simulink model "NLPIDVersion2"  (Simulink 7.3)
settings: Solver=ode5  StartTime=0.0  StopTime=inf  FixedStep=0.1  RelTol=1e-3
undefined symbols (not defined in the file): eta1_0_real, v1_0_real, velocitySatValues1
libraries: dspmtrx3 x16, simulink x14, dspindex x5, marine_gnc x4, simulink_extras x1, dspinverses x1
(part 1 of 4)
settings Model: Creator=Dinh  LastModifiedBy=mcl  BufferReuse=off
settings DataIOCC: LimitDataPoints=off  SaveOutput=off  SaveTime=off
settings OptimizationCC: BlockReduction=off  BooleanDataType=off  ConditionallyExecuteInputs=off  OptimizeBlockIOStorage=off  BufferReuse=off  ExpressionFolding=off  LocalBlockOutputs=off  SimCompilerOptimization=On
settings SFSimCC: SimBuildMode=sf_nonincremental_build
settings RTWCC: SystemTargetFile=nidll.tlc  TemplateMakefile=nidll_vc.tmf  Description=NI Real-Time Target for Release 2007b or later  ProcessScript=nidll_make_rtw_hook
settings STFCustomTargetCC: MatFileLogging=on  SystemTargetFile=nidll.tlc

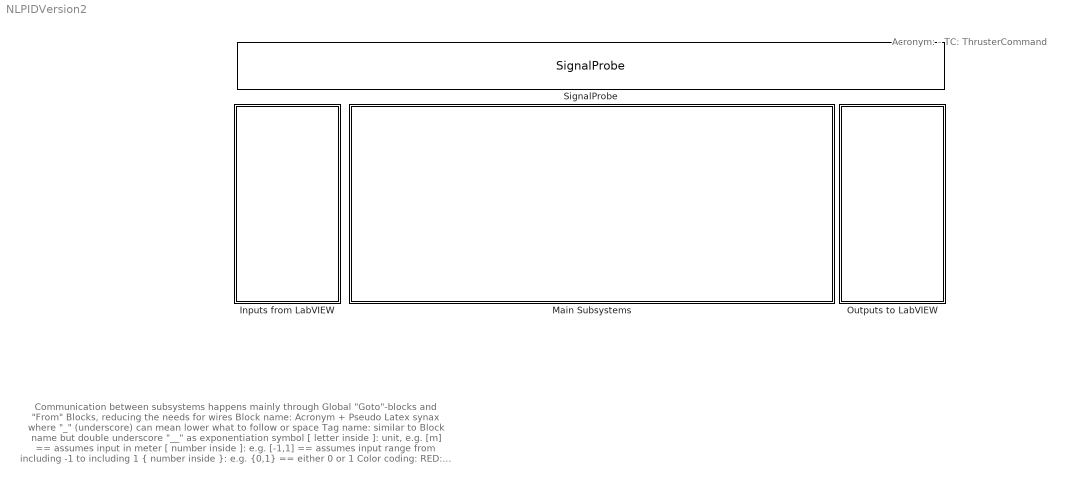
== system NLPIDVersion2 ==
  note: Communication between subsystems happens mainly through Global "Goto"-blocks and "From" Blocks,
      | reducing the needs for wires
      |
      | Block name: Acronym + Pseudo Latex synax where "_" (underscore) can mean lower what to follow or space
      | Tag name: similar to Block name but double underscore "__" as exponentiation symbol
      |
      | [ letter inside ]: unit, e.g. [m] == assumes input in meter
      | [ number inside ]: e.g. [-1,1] == assumes input range from including -1 to including 1
      | { number inside }:  e.g. {0,1} == either 0 or 1
      |
      | Color coding:
      | RED: Sinks (output ports, terminators, to workspace blocks, etc.)
      | GREEN Sources (inputs ports, constants, etc.)
      | CYAN: Memory blocks: Integrators, unit delays, memory, transfer functions, state space blocks, etc
      | GRAY: Logics blocks: Logic action ports, subsystem enable, etc.
      | ORANGE: GOTO blocks
      | MAGENTA: FROM blocks
      | YELLOW: All remaining blocks,
  note: Acronym:
      | - TC: ThrusterCommand
  Inputs from LabVIEW : Subsystem
  Main Subsystems : Subsystem
  Outputs to LabVIEW : Subsystem
  SignalProbe : S-Function  Description=Use this block with SIT.  FunctionName=SignalProbe  Parameters=1  EnableBusSupport=off
      settings: PreSaveFcn=NISIT_ModelVars;
      mask Description: The LabVIEW Simulation Interface Toolkit uses the SignalProbe block to probe the signals in the model. The SignalProbe block must be on the top level of the model hierarchy. You can have only one SignalProbe block per model file. Do not rename the SignalProbe block. Do not change the name of another model block to SignalProbe.

== system NLPIDVersion2/Inputs from LabVIEW ==
  Control Input Selector : Constant  Value=0
  Control Mode Selector : Constant  Value=0
  Enable CSE1 : Constant  Value=0
  Linear Simulator : Subsystem
  Path : Subsystem
  PlayStation3 : Subsystem
  Setpoint : Subsystem
  ctrl1: Dynamic Positioning : Subsystem
  ctrl2: LOS LgV backstepping II : Subsystem
  tag scope: controlInputSelector=global, controlModeSelector=global, enableCSE1=global
  wires:
  Control Mode Selector/1 -> [controlModeSelector]
  Control Input Selector/1 -> [controlInputSelector]
  Enable CSE1/1 -> [enableCSE1]

== system NLPIDVersion2/Main Subsystems ==
  C/S Enterprise 1 Matrices : Subsystem
  Control : Subsystem
  Data logging : Subsystem
  Guidance : Subsystem
  Naviagation : Subsystem
  Plant : Subsystem

== system NLPIDVersion2/Outputs to LabVIEW ==
  note: Gain blocks in this subsystem, functions as output ports for linking LabVIEW indicators through SIT Connection Manager
  Battery Voltage : Subsystem
  Command : Subsystem
  Mux9 : Mux  Inputs=2
  Naviagtion : Subsystem
  Visualization : Subsystem
  tag scope: eta_d=global
  wires:
  [pd] -> Mux9/1
  [psid] -> Mux9/2
  Mux9/1 -> [eta_d]

== system NLPIDVersion2/Inputs from LabVIEW/Linear Simulator ==
  note: Enable Linear Simulator: Activation
      | Reset Linear Simulator integrator: Reset
      | Initial u: Initial speed in surge
      | Initial v: Initial speed in sway
      | Initial r: Initial speed in yaw
      | Initial x: Initial position in surge
      | Initial y: Initial position in sway
      | Initial psi: Initial heading
  Enable Linear Simulator : Constant  Value=0
  Initial psi [rad] : Constant  Value=0  OutDataType=fixdt(1, 16)  OutScaling=2^0
  Initial r [rad/s] : Constant  Value=0  OutDataType=fixdt(1, 16)  OutScaling=2^0
  Initial u [m/s] : Constant  Value=0  OutDataType=fixdt(1, 16)  OutScaling=2^0
  Initial v [m/s] : Constant  Value=0  OutDataType=fixdt(1, 16)  OutScaling=2^0
  Initial x [m] : Constant  Value=0  OutDataType=fixdt(1, 16)  OutScaling=2^0
  Initial y [m] : Constant  Value=0  OutDataType=fixdt(1, 16)  OutScaling=2^0
  Mux : Mux  Inputs=3
  Mux1 : Mux  Inputs=3
  Reset Linear Simulator integrator : Constant  Value=0
  tag scope: LS_Enable=global, LS_Initial_eta=global, LS_Initial_nu=global, LS_Reset=global
  wires:
  Enable Linear Simulator/1 -> [LS_Enable]
  Reset Linear Simulator integrator/1 -> [LS_Reset]
  Mux/1 -> [LS_Initial_nu]
  Initial r [rad/s]/1 -> Mux/3
  Initial v [m/s]/1 -> Mux/2
  Initial u [m/s]/1 -> Mux/1
  Mux1/1 -> [LS_Initial_eta]
  Initial psi [rad]/1 -> Mux1/3
  Initial y [m]/1 -> Mux1/2
  Initial x [m]/1 -> Mux1/1

== system NLPIDVersion2/Inputs from LabVIEW/Path ==
  note: u_d: Desired surge speed of vessel
      | Path Selector: Workaround parameter for switching between linear path(==0) and ellipse path(==1)
      | x_dmax: Upper limit of desired x-ooordinate
      | x_dmin: Lower limit of desired x-coordiante
      | y_dmax: Upper limit of desired y-ooordinate
      | y_dmin: Lower limit of desired y-coordiante
      | Delta: Lookahead distance for LOS guidance
      | my: Gradient path minimizing tuning value
  Delta [m] : Constant  Value=2  OutDataType=fixdt(1, 16)  OutScaling=2^0
  Ellipse : Subsystem
  Linear : Subsystem
  Path Selector  [-] : Constant  Value=0
  my [-] : Constant  Value=10  OutDataType=fixdt(1, 16)  OutScaling=2^0
  u_d [m] : Constant  Value=0.15  OutDataType=fixdt(1, 16)  OutScaling=2^0
  x_dmax [m] : Constant  Value=40
  x_dmin [m] : Constant  Value=-40
  y_dmax [m] : Constant  Value=7
  y_dmin [m] : Constant  Value=-7
  tag scope: Delta=global, my=global, pathSelector=global, ud=global, xdmax=global, xdmin=global, ydmax=global, ydmin=global
  wires:
  u_d [m]/1 -> [ud]  "Desired speed [m/s]"
  Delta [m]/1 -> [Delta]  "Lookahead distance [m]"
  my [-]/1 -> [my]  "s tuning parameter"
  Path Selector  [-]/1 -> [pathSelector]  "chosen path {0,1}"
  x_dmax [m]/1 -> [xdmax]
  x_dmin [m]/1 -> [xdmin]
  y_dmax [m]/1 -> [ydmax]
  y_dmin [m]/1 -> [ydmin]

== system NLPIDVersion2/Inputs from LabVIEW/PlayStation3 ==
  note: Postive Y-axis of analog sticks points up (in the direction of the shoulder buttons)
      | Postive X-axis of analog sticks points to the right (in the direction of Triange, Circle, X and Square buttons)
      |
      | AS_LX: PS3 Analog Stick Left X-postition
      | AS_LY: PS3 Analog Stick Left Y-postition
      | AS_RX: PS3 Analog Stick Right X-postition
      | AS_RY: PS3 Analog Stick Right Y-postition
      | L2: PS3 bottom left sholderbutton
      | R2: PS3 bottom right shoulderbotton
      | PS3_BT_Power: PS3 command bow thruster power setpoint
      | PS3 _VSP_speed: PS3 command Voith Schneider Propeller speed
  "AS_LX [-] " : Constant  Value=0
  AS_LY [-] : Constant  Value=0
  AS_RX [-] : Constant  Value=0
  AS_RY [-] : Constant  Value=0
  L2 [-] : Constant  Value=0
  PS3_BT_Power  [-] : Constant  Value=0
  PS3_VSP_Speed  [-] : Constant  Value=0
  R2 [-] : Constant  Value=0
  ScalingLX : Gain  Gain=1/32767
  ScalingLY : Gain  Gain=1/32767
  ScalingRY : Gain  Gain=1/32767
  Scaling_RX : Gain  Gain=1/32767
  tag scope: PS3_AS_LX=global, PS3_AS_LY=global, PS3_AS_RX=global, PS3_AS_RY=global, PS3_BT_Power=global, PS3_L2=global, PS3_R2=global, PS3_VSP_Speed=global
  wires:
  PS3_VSP_Speed  [-]/1 -> [PS3_VSP_Speed]  "Voith Schnider Propeller Speed"
  PS3_BT_Power  [-]/1 -> [PS3_BT_Power]  "Bow Thruster Power"
  "AS_LX [-] "/1 -> ScalingLX/1  "x-position of left analog stick [-32767,32767]"
  ScalingLX/1 -> [PS3_AS_LX]  "x-position of left analog stick [-1,1]"
  AS_LY [-]/1 -> ScalingLY/1  "y-position of left analog stick [-32767,32767]"
  ScalingLY/1 -> [PS3_AS_LY]  "y-position of left analog stick [-1,1]"
  AS_RX [-]/1 -> Scaling_RX/1  "x-position of right analog stick  [-32767,32767]"
  Scaling_RX/1 -> [PS3_AS_RX]  "x-position of right analog stick  [-1,1]"
  ScalingRY/1 -> [PS3_AS_RY]  "y-position of right analog stick [-1,1]"
  AS_RY [-]/1 -> ScalingRY/1  "y-position of right analog stick [-32767,32767]"
  L2 [-]/1 -> [PS3_L2]  "L2 Button [-1,0]"
  R2 [-]/1 -> [PS3_R2]  "R2 Button [0,1]"

== system NLPIDVersion2/Inputs from LabVIEW/Setpoint ==
  Degrees to Radians : simulink_extras/Transformations/Degrees to Radians  SystemSampleTime=-1
  Mux : Mux  Inputs=3
  setpointpsi [deg] : Constant  Value=0
  setpointx [m] : Constant  Value=0
  setpointy [m] : Constant  Value=0
  tag scope: setpoint=global
  wires:
  Mux/1 -> [setpoint]
  setpointx [m]/1 -> Mux/1
  setpointy [m]/1 -> Mux/2
  setpointpsi [deg]/1 -> Degrees to Radians/1
  Degrees to Radians/1 -> Mux/3

== system NLPIDVersion2/Inputs from LabVIEW/ctrl1: Dynamic Positioning ==
  Kd : Subsystem
  Ki : Subsystem
  Kp : Subsystem
  "ctrl1 Reset Integrator " : Constant  Value=0
  ctrl1Kdpsi : Constant  Value=5
  ctrl1Kdx : Constant  Value=50
  ctrl1Kdy : Constant  Value=30
  ctrl1Kipsi : Constant  Value=0
  ctrl1Kix : Constant  Value=0
  ctrl1Kiy : Constant  Value=0
  ctrl1Kppsi : Constant  Value=0.5*3
  ctrl1Kpx : Constant  Value=2*1.5*2
  ctrl1Kpy : Constant  Value=2*10*2
  tag scope: ctrl1Reset=global
  wires:
  "ctrl1 Reset Integrator "/1 -> [ctrl1Reset]
  ctrl1Kpx/1 -> Kp/1(11)
  ctrl1Kpy/1 -> Kp/2(22)
  ctrl1Kppsi/1 -> Kp/3(33)
  ctrl1Kdx/1 -> Kd/1(11)
  ctrl1Kdy/1 -> Kd/2(22)
  ctrl1Kdpsi/1 -> Kd/3(33)
  ctrl1Kix/1 -> Ki/1(11)
  ctrl1Kiy/1 -> Ki/2(22)
  ctrl1Kipsi/1 -> Ki/3(33)

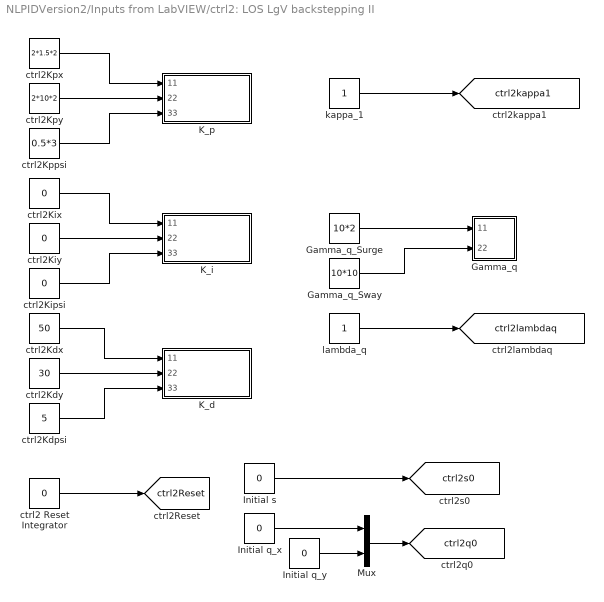
== system NLPIDVersion2/Inputs from LabVIEW/ctrl2: LOS LgV backstepping II ==
  Gamma_q : Subsystem
  Gamma_q_Surge : Constant  Value=10*2
  Gamma_q_Sway : Constant  Value=10*10
  Initial q_x : Constant  Value=0  OutDataType=fixdt(1, 16)  OutScaling=2^0
  Initial q_y : Constant  Value=0  OutDataType=fixdt(1, 16)  OutScaling=2^0
  Initial s : Constant  Value=0  OutDataType=fixdt(1, 16)  OutScaling=2^0
  K_d : Subsystem
  K_i : Subsystem
  K_p : Subsystem
  Mux : Mux  Inputs=2
  "ctrl2 Reset Integrator " : Constant  Value=0
  ctrl2Kdpsi : Constant  Value=5
  ctrl2Kdx : Constant  Value=50
  ctrl2Kdy : Constant  Value=30
  ctrl2Kipsi : Constant  Value=0
  ctrl2Kix : Constant  Value=0
  ctrl2Kiy : Constant  Value=0
  ctrl2Kppsi : Constant  Value=0.5*3
  ctrl2Kpx : Constant  Value=2*1.5*2
  ctrl2Kpy : Constant  Value=2*10*2
  kappa_1 : Constant
  lambda_q : Constant
  tag scope: ctrl2Reset=global, ctrl2kappa1=global, ctrl2lambdaq=global, ctrl2q0=global, ctrl2s0=global
  wires:
  ctrl2Kpx/1 -> K_p/1(11)
  ctrl2Kpy/1 -> K_p/2(22)
  ctrl2Kppsi/1 -> K_p/3(33)
  ctrl2Kdx/1 -> K_d/1(11)
  ctrl2Kdy/1 -> K_d/2(22)
  ctrl2Kdpsi/1 -> K_d/3(33)
  ctrl2Kix/1 -> K_i/1(11)
  ctrl2Kiy/1 -> K_i/2(22)
  ctrl2Kipsi/1 -> K_i/3(33)
  Gamma_q_Surge/1 -> Gamma_q/1(11)
  Gamma_q_Sway/1 -> Gamma_q/2(22)
  kappa_1/1 -> [ctrl2kappa1]
  lambda_q/1 -> [ctrl2lambdaq]
  Initial q_x/1 -> Mux/1
  Initial q_y/1 -> Mux/2
  Initial s/1 -> [ctrl2s0]
  Mux/1 -> [ctrl2q0]
  "ctrl2 Reset Integrator "/1 -> [ctrl2Reset]

== system NLPIDVersion2/Main Subsystems/C/S Enterprise 1 Matrices ==
  Inertia matrix : Subsystem
  Linear hydrodynamic dampning matrix : Subsystem
  Thruster configuration matrix : Subsystem
  tag scope: B=global, DL=global, M=global
  wires:
  Inertia matrix/1(M) -> [M]
  Linear hydrodynamic dampning matrix/1(D_L) -> [DL]
  Thruster configuration matrix/1(B) -> [B]

== system NLPIDVersion2/Main Subsystems/Control ==
  Control Switch : Subsystem
  DP control : Subsystem
  Nonlinear PID : Subsystem
  PS3 u input control : Subsystem
      settings: MinAlgLoopOccurrences=on
  Thruster allocation : Subsystem

== system NLPIDVersion2/Main Subsystems/Data logging ==
  note: Data logging:
      | - Create a file named CSE1_data.mat in CRIO
      | - Top row contains timestamp run-time
      | Rows contain values of the vector sent into the block at timestamp
      | -Row 1: Time since simulation start
      | -Row 2: Selected navigation system, 0 == QS, 1 == LS
      | -Row 3: Error signal from Qualisys
      | -Row 4: Residual from Qualisys
      | -Row 5 to 7: etadot, col ( xdot, ydot, psidot)
      | -Row 8 to 10: eta, col (x, y, psi)
      | -Row 11 to 13: nu, col (u, v, r)
      | -Row 14 to 16: DP eta_d, col(x_d_DP, y_d_DP, psi_d_DP)
      | -Row 17 to 19: chi, col( q_x, q_y, psi_los)
      | -Row 20: Selected path, 0 == Ellipse, 1 = Linear
      | -Row 21 to 23: Path eta_d, col(x_d_path, y_d_path, psi_d_path)
      | -Row 24: u_d
      | -Row: 25: v_s
      | -Row 26: s
      | -Row 27: Selected control system
      | -Row 28 to 34: thruster setting, ( u_1, u_2, u_3, u_4. u_5, BT_limit, VSP_limit)
      | -Row 35 to 37: tau, col( X, Y, N)
      | -Row 38 to 39: omega_qx, omega_qy
  Mux2 : Mux  Inputs=17
  To File : ToFile  Filename=Template_data.mat  MatrixName=Template_data
  wires:
  Mux2/1 -> To File/1
  [controlInputSelector] -> Mux2/1
  [QTM_Error] -> Mux2/2
  [QTM_Residual] -> Mux2/3
  [etadot] -> Mux2/4
  [eta] -> Mux2/5
  [nu] -> Mux2/6
  [setpoint] -> Mux2/7
  [chi] -> Mux2/8
  [pathSelector] -> Mux2/9
  [eta_d] -> Mux2/10
  [ud] -> Mux2/11
  [vs] -> Mux2/12
  [s] -> Mux2/13
  [controlModeSelector] -> Mux2/14
  [ThrusterSetting] -> Mux2/15
  [tau] -> Mux2/16
  [omegaq] -> Mux2/17

== system NLPIDVersion2/Main Subsystems/Guidance ==
  Line-Of-Sight Path-Following : Subsystem

== system NLPIDVersion2/Main Subsystems/Naviagation ==
  Input from SIT : Subsystem
  Navigation Switch : Subsystem

== system NLPIDVersion2/Main Subsystems/Plant ==
  CSE1 actuator : Subsystem
  Inverse : Product  Inputs=/  Multiplication=Matrix(*)
  Linear Simulator : Subsystem
      settings: MinAlgLoopOccurrences=on
  Thruster setting workaround : Subsystem
  saturation : Subsystem
  tag scope: LS_eta=global, LS_etadot=global, LS_nu=global
  wires:
  [enableCSE1] -> CSE1 actuator/Enable
  [LS_Enable] -> Linear Simulator/Enable
  saturation/1(sat_tau) -> Linear Simulator/1(tau)
  [tau] -> saturation/1(tau)
  Linear Simulator/1(eta_hil) -> [LS_eta]
  Linear Simulator/2(nu_hil) -> [LS_nu]
  Linear Simulator/3(etadot_hil) -> [LS_etadot]
  [M] -> Inverse/1
  Inverse/1 -> Linear Simulator/2(M_inv)
  [DL] -> Linear Simulator/3(D_L)
  [LS_Reset] -> Linear Simulator/4(Reset)
  [LS_Initial_eta] -> Linear Simulator/5(eta_0)
  [LS_Initial_nu] -> Linear Simulator/6(nu_0)
  [TC] -> Thruster setting workaround/1(TC)
  [ThrusterSetting] -> CSE1 actuator/1(Thurster setting)

== system NLPIDVersion2/Outputs to LabVIEW/Battery Voltage ==
  note: Main battery is multipled by 2, since the voltage is halfed at measuring point
  Battery Bow Thruster : Gain  ParameterDataType=fixdt(1, 16)  ParameterScaling=2^0  OutDataType=fixdt(1, 16)  OutScaling=2^0
  Battery Main : Gain  Gain=2  ParameterDataType=fixdt(1, 16)  ParameterScaling=2^0  OutDataType=fixdt(1, 16)  OutScaling=2^0
  Battery Servo : Gain  ParameterDataType=fixdt(1, 16)  ParameterScaling=2^0  OutDataType=fixdt(1, 16)  OutScaling=2^0
  Terminator Bow Thruster Battery : Terminator
  Terminator Main Battery : Terminator
  Terminator Servo Battery : Terminator
  wires:
  [Battery_BT] -> Battery Bow Thruster/1
  Battery Bow Thruster/1 -> Terminator Bow Thruster Battery/1
  [Battery_Servo] -> Battery Servo/1
  Battery Servo/1 -> Terminator Servo Battery/1
  [Battery_Main] -> Battery Main/1
  Battery Main/1 -> Terminator Main Battery/1

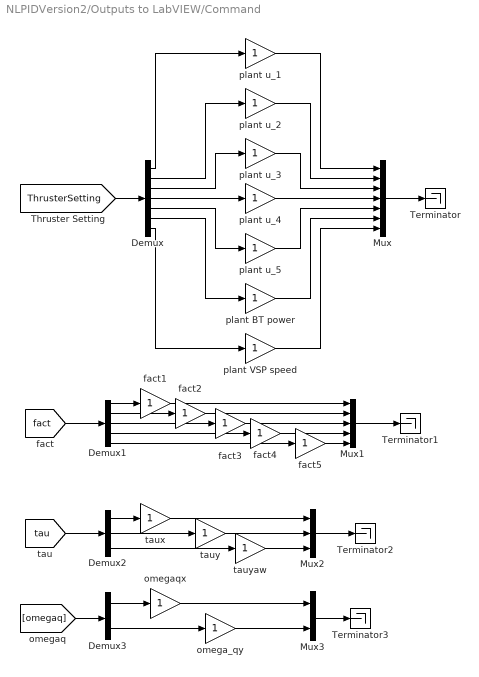
== system NLPIDVersion2/Outputs to LabVIEW/Command ==
  Demux : Demux  Outputs=7
  Demux1 : Demux  Outputs=5
  Demux2 : Demux  Outputs=3
  Demux3 : Demux  Outputs=2
  Mux : Mux  Inputs=7
  Mux1 : Mux  Inputs=5
  Mux2 : Mux  Inputs=3
  Mux3 : Mux  Inputs=2
  Terminator{,1..3} (4 alike) : Terminator
  fact{1..5} (5 alike) : Gain  ParameterDataType=fixdt(1, 16)  ParameterScaling=2^0  OutDataType=fixdt(1, 16)  OutScaling=2^0
  omega_qy : Gain  ParameterDataType=fixdt(1, 16)  ParameterScaling=2^0  OutDataType=fixdt(1, 16)  OutScaling=2^0
  omegaqx : Gain  ParameterDataType=fixdt(1, 16)  ParameterScaling=2^0  OutDataType=fixdt(1, 16)  OutScaling=2^0
  plant BT power : Gain  ParameterDataType=fixdt(1, 16)  ParameterScaling=2^0  OutDataType=fixdt(1, 16)  OutScaling=2^0
  plant VSP speed : Gain  ParameterDataType=fixdt(1, 16)  ParameterScaling=2^0  OutDataType=fixdt(1, 16)  OutScaling=2^0
  plant u_{1..5} (5 alike) : Gain  ParameterDataType=fixdt(1, 16)  ParameterScaling=2^0  OutDataType=fixdt(1, 16)  OutScaling=2^0
  taux : Gain  ParameterDataType=fixdt(1, 16)  ParameterScaling=2^0  OutDataType=fixdt(1, 16)  OutScaling=2^0
  tauy : Gain  ParameterDataType=fixdt(1, 16)  ParameterScaling=2^0  OutDataType=fixdt(1, 16)  OutScaling=2^0
  tauyaw : Gain  ParameterDataType=fixdt(1, 16)  ParameterScaling=2^0  OutDataType=fixdt(1, 16)  OutScaling=2^0
  wires:
  Demux/1 -> plant u_1/1
  Demux/2 -> plant u_2/1
  Demux/3 -> plant u_3/1
  Demux/4 -> plant u_4/1
  plant u_4/1 -> Mux/4
  plant u_1/1 -> Mux/1
  plant u_2/1 -> Mux/2
  plant u_3/1 -> Mux/3
  Demux/5 -> plant u_5/1
  Demux/6 -> plant BT power/1
  Demux/7 -> plant VSP speed/1
  plant u_5/1 -> Mux/5
  plant BT power/1 -> Mux/6
  plant VSP speed/1 -> Mux/7
  Mux/1 -> Terminator/1
  [ThrusterSetting] -> Demux/1
  fact1/1 -> Mux1/1
  fact2/1 -> Mux1/2
  fact3/1 -> Mux1/3
  fact4/1 -> Mux1/4
  fact5/1 -> Mux1/5
  Demux1/1 -> fact1/1
  Demux1/2 -> fact2/1
  Demux1/3 -> fact3/1
  Demux1/4 -> fact4/1
  Demux1/5 -> fact5/1
  [fact] -> Demux1/1
  Demux2/1 -> taux/1
  Demux2/2 -> tauy/1
  Demux2/3 -> tauyaw/1
  taux/1 -> Mux2/1
  tauy/1 -> Mux2/2
  tauyaw/1 -> Mux2/3
  Mux1/1 -> Terminator1/1
  Mux2/1 -> Terminator2/1
  [tau] -> Demux2/1
  Demux3/1 -> omegaqx/1
  Demux3/2 -> omega_qy/1
  omegaqx/1 -> Mux3/1
  omega_qy/1 -> Mux3/2
  Mux3/1 -> Terminator3/1
  [omegaq] -> Demux3/1

== system NLPIDVersion2/Outputs to LabVIEW/Naviagtion ==
  CSE1_r [deg/s] : Gain  Gain=180/pi  ParameterDataType=fixdt(1, 16)  ParameterScaling=2^0  OutDataType=fixdt(1, 16)  OutScaling=2^0
  CSE1_u [m/s] : Gain  ParameterDataType=fixdt(1, 16)  ParameterScaling=2^0  OutDataType=fixdt(1, 16)  OutScaling=2^0
  CSE1_v [m/s] : Gain  ParameterDataType=fixdt(1, 16)  ParameterScaling=2^0  OutDataType=fixdt(1, 16)  OutScaling=2^0
  Demux4 : Demux  Outputs=3
  Mux4 : Mux  Inputs=3
  Terminator3 : Terminator
  wires:
  CSE1_v [m/s]/1 -> Mux4/2
  CSE1_r [deg/s]/1 -> Mux4/3
  CSE1_u [m/s]/1 -> Mux4/1
  Demux4/3 -> CSE1_r [deg/s]/1
  Demux4/2 -> CSE1_v [m/s]/1
  Demux4/1 -> CSE1_u [m/s]/1
  Mux4/1 -> Terminator3/1
  [nu] -> Demux4/1

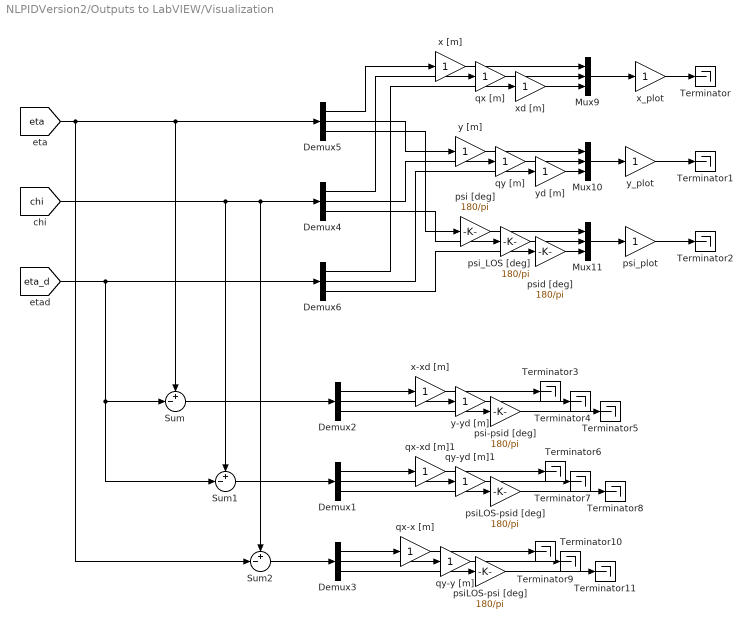
== system NLPIDVersion2/Outputs to LabVIEW/Visualization ==
  Demux{1..6} (6 alike) : Demux  Outputs=3
  Mux10 : Mux  Inputs=3
  Mux11 : Mux  Inputs=3
  Mux9 : Mux  Inputs=3
  Sum : Sum  Inputs=+-|  OutDataType=fixdt(1, 16)  OutScaling=2^0
  Sum1 : Sum  Inputs=+-|  OutDataType=fixdt(1, 16)  OutScaling=2^0
  Sum2 : Sum  Inputs=+-|  OutDataType=fixdt(1, 16)  OutScaling=2^0
  Terminator{,1..11} (12 alike) : Terminator
  psi [deg] : Gain  Gain=180/pi  ParameterDataType=fixdt(1, 16)  ParameterScaling=2^0  OutDataType=fixdt(1, 16)  OutScaling=2^0
  psi-psid [deg] : Gain  Gain=180/pi  ParameterDataType=fixdt(1, 16)  ParameterScaling=2^0  OutDataType=fixdt(1, 16)  OutScaling=2^0
  psiLOS-psi [deg] : Gain  Gain=180/pi  ParameterDataType=fixdt(1, 16)  ParameterScaling=2^0  OutDataType=fixdt(1, 16)  OutScaling=2^0
  psiLOS-psid [deg] : Gain  Gain=180/pi  ParameterDataType=fixdt(1, 16)  ParameterScaling=2^0  OutDataType=fixdt(1, 16)  OutScaling=2^0
  psi_LOS [deg] : Gain  Gain=180/pi  ParameterDataType=fixdt(1, 16)  ParameterScaling=2^0  OutDataType=fixdt(1, 16)  OutScaling=2^0
  psi_plot : Gain  ParameterDataType=fixdt(1, 16)  ParameterScaling=2^0  OutDataType=fixdt(1, 16)  OutScaling=2^0
  psid [deg] : Gain  Gain=180/pi  ParameterDataType=fixdt(1, 16)  ParameterScaling=2^0  OutDataType=fixdt(1, 16)  OutScaling=2^0
  qx [m] : Gain  ParameterDataType=fixdt(1, 16)  ParameterScaling=2^0  OutDataType=fixdt(1, 16)  OutScaling=2^0
  qx-x [m] : Gain  ParameterDataType=fixdt(1, 16)  ParameterScaling=2^0  OutDataType=fixdt(1, 16)  OutScaling=2^0
  qx-xd [m]1 : Gain  ParameterDataType=fixdt(1, 16)  ParameterScaling=2^0  OutDataType=fixdt(1, 16)  OutScaling=2^0
  qy [m] : Gain  ParameterDataType=fixdt(1, 16)  ParameterScaling=2^0  OutDataType=fixdt(1, 16)  OutScaling=2^0
  qy-y [m] : Gain  ParameterDataType=fixdt(1, 16)  ParameterScaling=2^0  OutDataType=fixdt(1, 16)  OutScaling=2^0
  qy-yd [m]1 : Gain  ParameterDataType=fixdt(1, 16)  ParameterScaling=2^0  OutDataType=fixdt(1, 16)  OutScaling=2^0
  x [m] : Gain  ParameterDataType=fixdt(1, 16)  ParameterScaling=2^0  OutDataType=fixdt(1, 16)  OutScaling=2^0
  x-xd [m] : Gain  ParameterDataType=fixdt(1, 16)  ParameterScaling=2^0  OutDataType=fixdt(1, 16)  OutScaling=2^0
  x_plot : Gain  ParameterDataType=fixdt(1, 16)  ParameterScaling=2^0  OutDataType=fixdt(1, 16)  OutScaling=2^0
  xd [m] : Gain  ParameterDataType=fixdt(1, 16)  ParameterScaling=2^0  OutDataType=fixdt(1, 16)  OutScaling=2^0
  y [m] : Gain  ParameterDataType=fixdt(1, 16)  ParameterScaling=2^0  OutDataType=fixdt(1, 16)  OutScaling=2^0
  y-yd [m] : Gain  ParameterDataType=fixdt(1, 16)  ParameterScaling=2^0  OutDataType=fixdt(1, 16)  OutScaling=2^0
  y_plot : Gain  ParameterDataType=fixdt(1, 16)  ParameterScaling=2^0  OutDataType=fixdt(1, 16)  OutScaling=2^0
  yd [m] : Gain  ParameterDataType=fixdt(1, 16)  ParameterScaling=2^0  OutDataType=fixdt(1, 16)  OutScaling=2^0
  wires:
  Demux5/1 -> x [m]/1
  Demux4/1 -> qx [m]/1
  Demux6/1 -> xd [m]/1
  Demux5/2 -> y [m]/1
  Demux4/2 -> qy [m]/1
  Demux6/2 -> yd [m]/1
  Demux5/3 -> psi [deg]/1
  Demux4/3 -> psi_LOS [deg]/1
  Demux6/3 -> psid [deg]/1
  Mux9/1 -> x_plot/1
  Mux10/1 -> y_plot/1
  Mux11/1 -> psi_plot/1
  x_plot/1 -> Terminator/1
  x [m]/1 -> Mux9/1
  qx [m]/1 -> Mux9/2
  xd [m]/1 -> Mux9/3
  y [m]/1 -> Mux10/1
  qy [m]/1 -> Mux10/2
  yd [m]/1 -> Mux10/3
  psi [deg]/1 -> Mux11/1
  psi_LOS [deg]/1 -> Mux11/2
  psid [deg]/1 -> Mux11/3
  y_plot/1 -> Terminator1/1
  psi_plot/1 -> Terminator2/1
  [eta] -> Demux5/1, Sum/1, Sum2/2
  [chi] -> Sum1/1, Demux4/1, Sum2/1
  [eta_d] -> Demux6/1, Sum/2, Sum1/2
  Sum/1 -> Demux2/1
  Sum1/1 -> Demux1/1
  Sum2/1 -> Demux3/1
  Demux2/1 -> x-xd [m]/1
  Demux2/2 -> y-yd [m]/1
  Demux2/3 -> psi-psid [deg]/1
  Demux1/1 -> qx-xd [m]1/1
  Demux1/2 -> qy-yd [m]1/1
  Demux1/3 -> psiLOS-psid [deg]/1
  Demux3/2 -> qy-y [m]/1
  Demux3/3 -> psiLOS-psi [deg]/1
  Demux3/1 -> qx-x [m]/1
  x-xd [m]/1 -> Terminator3/1
  y-yd [m]/1 -> Terminator4/1
  psi-psid [deg]/1 -> Terminator5/1
  qy-yd [m]1/1 -> Terminator7/1
  psiLOS-psid [deg]/1 -> Terminator8/1
  qx-xd [m]1/1 -> Terminator6/1
  qy-y [m]/1 -> Terminator10/1
  psiLOS-psi [deg]/1 -> Terminator11/1
  qx-x [m]/1 -> Terminator9/1

== system NLPIDVersion2/Inputs from LabVIEW/Path/Ellipse ==
  note: origin_x: ellipse origin x-coordinate
      | origin_y: ellipse origin y-coordinate
      | r_x: ellipse radius x-direction
      | r_y: ellipse radius y-direction
      | k: step scaling factor of path parameter
  k [-] : Constant  Value=pi/180*2  OutDataType=fixdt(1, 16)  OutScaling=2^0
  r_x [m] : Constant  Value=5.5  OutDataType=fixdt(1, 16)  OutScaling=2^0
  r_y [m] : Constant  Value=2  OutDataType=fixdt(1, 16)  OutScaling=2^0
  x_0 [m] : Constant  Value=4.5  OutDataType=fixdt(1, 16)  OutScaling=2^0
  y_0 [m] : Constant  Value=0  OutDataType=fixdt(1, 16)  OutScaling=2^0
  tag scope: k=global, rx=global, ry=global, x0=global, y0=global
  wires:
  x_0 [m]/1 -> [x0]  "x-coord. origin ellipse path [m]"
  y_0 [m]/1 -> [y0]  "y-coord. origin ellipse path [m]"
  r_x [m]/1 -> [rx]  "radius ellipse path x-axis [m]"
  r_y [m]/1 -> [ry]  "radius ellipse path y-axis [m]"
  k [-]/1 -> [k]  "step scaling factor ellipse path [-]"

== system NLPIDVersion2/Inputs from LabVIEW/Path/Linear ==
  note: x_1: reference way-point x-coordinate
      | y_1: reference way-point y-coordinate
      | x_2: direction way-point x-coordinate
      | y_2: direction way-point y-coordinate
  x_1 [m] : Constant  Value=0  OutDataType=fixdt(1, 16)  OutScaling=2^0
  x_2 [m] : Constant  Value=5.5  OutDataType=fixdt(1, 16)  OutScaling=2^0
  y_1 [m] : Constant  Value=0  OutDataType=fixdt(1, 16)  OutScaling=2^0
  y_2 [m] : Constant  Value=2  OutDataType=fixdt(1, 16)  OutScaling=2^0
  tag scope: x1=global, x2=global, y1=global, y2=global
  wires:
  x_1 [m]/1 -> [x1]  "x-coord. reference point path [m]"
  y_1 [m]/1 -> [y1]  "y-coord, reference point path [m]"
  x_2 [m]/1 -> [x2]  "x-coord, direction point path [m]"
  y_2 [m]/1 -> [y2]  "y-coord, direction point path [m]"

== system NLPIDVersion2/Inputs from LabVIEW/ctrl1: Dynamic Positioning/Kd ==
  note: Creating 3x3 diagonal matrix
  11 : Inport
  22 : Inport  Port=2
  33 : Inport  Port=3
  {12..13,21,23,31..32} (6 alike) : Constant  Value=0
  Mux : Mux  Inputs=9
  "[3x3]" : Reshape  OutputDimensionality=Customize  OutputDimensions=[3,3]
  tag scope: ctrl1Kd=global
  wires:
  "[3x3]"/1 -> [ctrl1Kd]
  33/1 -> Mux/9
  23/1 -> Mux/8
  13/1 -> Mux/7
  32/1 -> Mux/6
  22/1 -> Mux/5
  12/1 -> Mux/4
  31/1 -> Mux/3
  21/1 -> Mux/2
  11/1 -> Mux/1
  Mux/1 -> "[3x3]"/1

== system NLPIDVersion2/Inputs from LabVIEW/ctrl1: Dynamic Positioning/Ki ==
  note: Creating 3x3 diagonal matrix
  11 : Inport
  22 : Inport  Port=2
  33 : Inport  Port=3
  {12..13,21,23,31..32} (6 alike) : Constant  Value=0
  Mux : Mux  Inputs=9
  "[3x3]" : Reshape  OutputDimensionality=Customize  OutputDimensions=[3,3]
  tag scope: ctrl1Ki=global
  wires:
  "[3x3]"/1 -> [ctrl1Ki]
  33/1 -> Mux/9
  23/1 -> Mux/8
  13/1 -> Mux/7
  32/1 -> Mux/6
  22/1 -> Mux/5
  12/1 -> Mux/4
  31/1 -> Mux/3
  21/1 -> Mux/2
  11/1 -> Mux/1
  Mux/1 -> "[3x3]"/1

== system NLPIDVersion2/Inputs from LabVIEW/ctrl1: Dynamic Positioning/Kp ==
  note: Creating 3x3 diagonal matrix
  11 : Inport
  22 : Inport  Port=2
  33 : Inport  Port=3
  {12..13,21,23,31..32} (6 alike) : Constant  Value=0
  Mux : Mux  Inputs=9
  "[3x3]" : Reshape  OutputDimensionality=Customize  OutputDimensions=[3,3]
  tag scope: ctrl1Kp=global
  wires:
  Mux/1 -> "[3x3]"/1
  11/1 -> Mux/1
  21/1 -> Mux/2
  31/1 -> Mux/3
  12/1 -> Mux/4
  22/1 -> Mux/5
  32/1 -> Mux/6
  13/1 -> Mux/7
  23/1 -> Mux/8
  33/1 -> Mux/9
  "[3x3]"/1 -> [ctrl1Kp]

== system NLPIDVersion2/Inputs from LabVIEW/ctrl2: LOS LgV backstepping II/Gamma_q ==
  11 : Inport
  22 : Inport  Port=2
  12 : Constant  Value=0
  21 : Constant  Value=0
  Mux : Mux
  "[2x2]" : Reshape  OutputDimensionality=Customize  OutputDimensions=[2,2]
  tag scope: ctrl2Gammaq=global
  wires:
  Mux/1 -> "[2x2]"/1
  11/1 -> Mux/1
  21/1 -> Mux/2
  12/1 -> Mux/3
  22/1 -> Mux/4
  "[2x2]"/1 -> [ctrl2Gammaq]

== system NLPIDVersion2/Inputs from LabVIEW/ctrl2: LOS LgV backstepping II/K_d ==
  note: Creating 3x3 diagonal matrix
  11 : Inport
  22 : Inport  Port=2
  33 : Inport  Port=3
  {12..13,21,23,31..32} (6 alike) : Constant  Value=0
  Mux : Mux  Inputs=9
  "[3x3]" : Reshape  OutputDimensionality=Customize  OutputDimensions=[3,3]
  tag scope: ctrl2Kd=global
  wires:
  "[3x3]"/1 -> [ctrl2Kd]
  33/1 -> Mux/9
  23/1 -> Mux/8
  13/1 -> Mux/7
  32/1 -> Mux/6
  22/1 -> Mux/5
  12/1 -> Mux/4
  31/1 -> Mux/3
  21/1 -> Mux/2
  11/1 -> Mux/1
  Mux/1 -> "[3x3]"/1

== system NLPIDVersion2/Inputs from LabVIEW/ctrl2: LOS LgV backstepping II/K_i ==
  note: Creating 3x3 diagonal matrix
  11 : Inport
  22 : Inport  Port=2
  33 : Inport  Port=3
  {12..13,21,23,31..32} (6 alike) : Constant  Value=0
  Mux : Mux  Inputs=9
  "[3x3]" : Reshape  OutputDimensionality=Customize  OutputDimensions=[3,3]
  tag scope: ctrl2Ki=global
  wires:
  "[3x3]"/1 -> [ctrl2Ki]
  33/1 -> Mux/9
  23/1 -> Mux/8
  13/1 -> Mux/7
  32/1 -> Mux/6
  22/1 -> Mux/5
  12/1 -> Mux/4
  31/1 -> Mux/3
  21/1 -> Mux/2
  11/1 -> Mux/1
  Mux/1 -> "[3x3]"/1

== system NLPIDVersion2/Inputs from LabVIEW/ctrl2: LOS LgV backstepping II/K_p ==
  note: Creating 3x3 diagonal matrix
  11 : Inport
  22 : Inport  Port=2
  33 : Inport  Port=3
  {12..13,21,23,31..32} (6 alike) : Constant  Value=0
  Mux : Mux  Inputs=9
  "[3x3]" : Reshape  OutputDimensionality=Customize  OutputDimensions=[3,3]
  tag scope: ctrl2Kp=global
  wires:
  Mux/1 -> "[3x3]"/1
  11/1 -> Mux/1
  21/1 -> Mux/2
  31/1 -> Mux/3
  12/1 -> Mux/4
  22/1 -> Mux/5
  32/1 -> Mux/6
  13/1 -> Mux/7
  23/1 -> Mux/8
  33/1 -> Mux/9
  "[3x3]"/1 -> [ctrl2Kp]

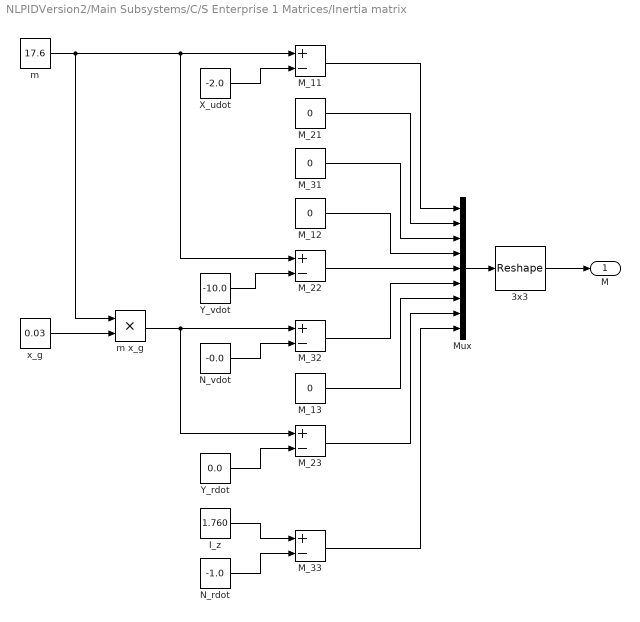
== system NLPIDVersion2/Main Subsystems/C/S Enterprise 1 Matrices/Inertia matrix ==
  3x3 : Reshape  OutputDimensionality=Customize  OutputDimensions=[3,3]
  I_z : Constant  Value=1.760
  M_{11,22..23,32..33} (5 alike) : Sum  Inputs=+-
  M_{12..13,21,31} (4 alike) : Constant  Value=0
  Mux : Mux  Inputs=9
  N_rdot : Constant  Value=-1.0
  N_vdot : Constant  Value=-0.0
  X_udot : Constant  Value=-2.0
  Y_rdot : Constant  Value=0.0
  Y_vdot : Constant  Value=-10.0
  m : Constant  Value=17.6
  m x_g : Product  RndMeth=Zero
  x_g : Constant  Value=0.03
  M : Outport
  wires:
  3x3/1 -> M/1
  Mux/1 -> 3x3/1
  M_33/1 -> Mux/9
  M_23/1 -> Mux/8
  M_13/1 -> Mux/7
  M_32/1 -> Mux/6
  M_22/1 -> Mux/5
  M_12/1 -> Mux/4
  M_31/1 -> Mux/3
  M_21/1 -> Mux/2
  M_11/1 -> Mux/1
  N_rdot/1 -> M_33/2
  I_z/1 -> M_33/1
  Y_rdot/1 -> M_23/2
  N_vdot/1 -> M_32/2
  m x_g/1 -> M_23/1, M_32/1
  x_g/1 -> m x_g/2
  Y_vdot/1 -> M_22/2
  X_udot/1 -> M_11/2
  m/1 -> m x_g/1, M_22/1, M_11/1

== system NLPIDVersion2/Main Subsystems/C/S Enterprise 1 Matrices/Linear hydrodynamic dampning matrix ==
  -N_r : Gain  Gain=-1  ParameterDataType=fixdt(1, 16)  ParameterScaling=2^0  OutDataType=fixdt(1, 16)  OutScaling=2^0
  -N_v : Gain  Gain=-1  ParameterDataType=fixdt(1, 16)  ParameterScaling=2^0  OutDataType=fixdt(1, 16)  OutScaling=2^0
  -X_u : Gain  Gain=-1  ParameterDataType=fixdt(1, 16)  ParameterScaling=2^0  OutDataType=fixdt(1, 16)  OutScaling=2^0
  -Y_v : Gain  Gain=-1  ParameterDataType=fixdt(1, 16)  ParameterScaling=2^0  OutDataType=fixdt(1, 16)  OutScaling=2^0
  -Y_vr : Gain  Gain=-1  ParameterDataType=fixdt(1, 16)  ParameterScaling=2^0  OutDataType=fixdt(1, 16)  OutScaling=2^0
  D_L_{12..13,21,31} (4 alike) : Constant  Value=0
  Linear Dampning matrix : Reshape  OutputDimensionality=Customize  OutputDimensions=[3,3]
  Mux : Mux  Inputs=9
  N_r : Constant  Value=-1.900
  N_v : Constant  Value=0.18140
  X_u : Constant  Value=-0.59739
  Y_r : Constant  Value=-7.250
  Y_v : Constant  Value=-3.50625
  D_L : Outport
  wires:
  -N_r/1 -> Mux/9
  -Y_vr/1 -> Mux/8
  D_L_13/1 -> Mux/7
  -N_v/1 -> Mux/6
  -Y_v/1 -> Mux/5
  D_L_12/1 -> Mux/4
  D_L_31/1 -> Mux/3
  D_L_21/1 -> Mux/2
  -X_u/1 -> Mux/1
  N_r/1 -> -N_r/1
  Y_r/1 -> -Y_vr/1
  N_v/1 -> -N_v/1
  Y_v/1 -> -Y_v/1
  Linear Dampning matrix/1 -> D_L/1
  Mux/1 -> Linear Dampning matrix/1
  X_u/1 -> -X_u/1

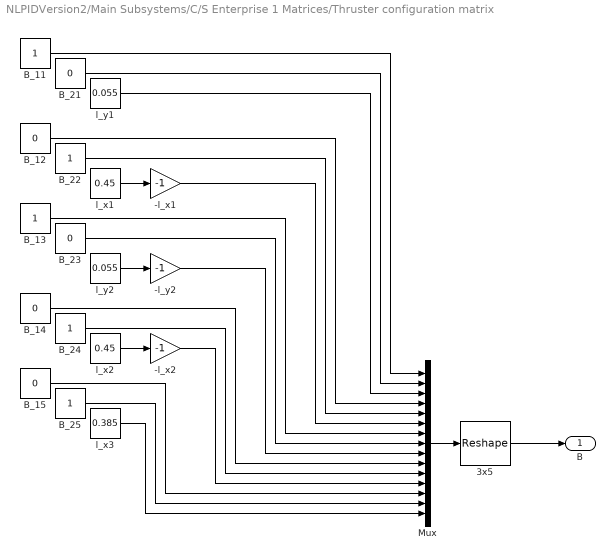
== system NLPIDVersion2/Main Subsystems/C/S Enterprise 1 Matrices/Thruster configuration matrix ==
  -l_x1 : Gain  Gain=-1
  -l_x2 : Gain  Gain=-1
  -l_y2 : Gain  Gain=-1
  3x5 : Reshape  OutputDimensionality=Customize  OutputDimensions=[3,5]
  B_{11,13,22,24..25} (5 alike) : Constant
  B_{12,14..15,21,23} (5 alike) : Constant  Value=0
  Mux : Mux  Inputs=15
  l_x1 : Constant  Value=0.45
  l_x2 : Constant  Value=0.45
  l_x3 : Constant  Value=0.385
  l_y1 : Constant  Value=0.055
  l_y2 : Constant  Value=0.055
  B : Outport
  wires:
  l_x3/1 -> Mux/15
  B_25/1 -> Mux/14
  B_15/1 -> Mux/13
  -l_x2/1 -> Mux/12
  -l_y2/1 -> Mux/9
  -l_x1/1 -> Mux/6
  l_x2/1 -> -l_x2/1
  B_24/1 -> Mux/11
  B_14/1 -> Mux/10
  l_y2/1 -> -l_y2/1
  B_23/1 -> Mux/8
  B_13/1 -> Mux/7
  l_x1/1 -> -l_x1/1
  B_22/1 -> Mux/5
  B_12/1 -> Mux/4
  l_y1/1 -> Mux/3
  B_21/1 -> Mux/2
  B_11/1 -> Mux/1
  3x5/1 -> B/1
  Mux/1 -> 3x5/1

== system NLPIDVersion2/Main Subsystems/Control/Control Switch ==
  note: 0 - PS3 u input control
      | 1 - DP control
      | 2 - LgV2 control
  tau Switch : MultiPortSwitch  zeroidx=on
  tag scope: tau=global
  wires:
  [controlModeSelector] -> tau Switch/1
  tau Switch/1 -> [tau]
  [PS3tau] -> tau Switch/2
  [ctrl1tau] -> tau Switch/3
  [ctrl2tau] -> tau Switch/4

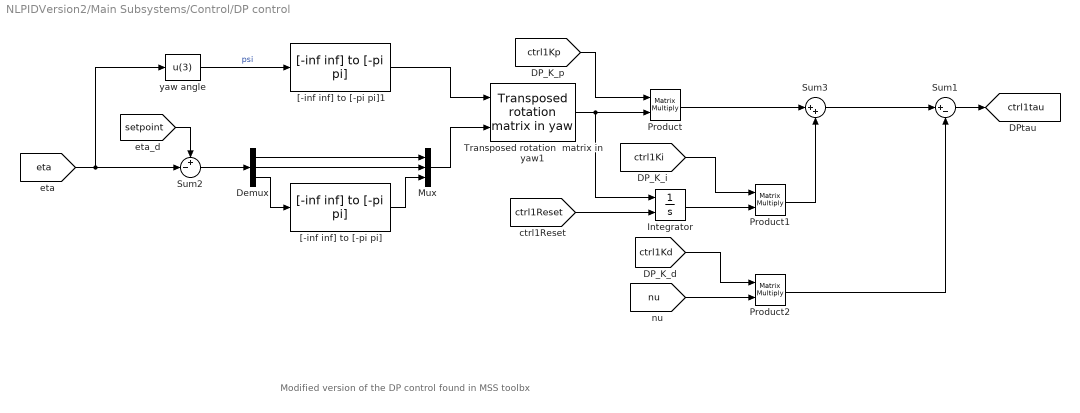
== system NLPIDVersion2/Main Subsystems/Control/DP control ==
  note: Modified version of the DP control found in MSS toolbx
  Demux : Demux  Outputs=3
  Integrator : Integrator  ExternalReset=level
  Mux : Mux  Inputs=3
  Product : Product  Multiplication=Matrix(*)  OutDataType=fixdt(1, 16)  OutScaling=2^0  RndMeth=Zero
  Product1 : Product  Multiplication=Matrix(*)  OutDataType=fixdt(1, 16)  OutScaling=2^0  RndMeth=Zero
  Product2 : Product  Multiplication=Matrix(*)  OutDataType=fixdt(1, 16)  OutScaling=2^0  RndMeth=Zero
  Sum1 : Sum  Inputs=|+-  SaturateOnIntegerOverflow=on  InputSameDT=on  OutDataTypeStr=Inherit: Same as first input
  Sum2 : Sum  Inputs=+-|  SaturateOnIntegerOverflow=on  InputSameDT=on  OutDataTypeStr=Inherit: Same as first input
  Sum3 : Sum  Inputs=|++  SaturateOnIntegerOverflow=on  InputSameDT=on  OutDataTypeStr=Inherit: Same as first input
  Transposed rotation  matrix in yaw1 : marine_gnc/Models/ Kinematics/Transposed rotation  matrix in yaw  SystemSampleTime=-1
  "[-inf inf] to [-pi pi]" : marine_gnc/Utilities/Math Operations/[-inf inf] to [-pi pi]  SystemSampleTime=-1
  "[-inf inf] to [-pi pi]1" : marine_gnc/Utilities/Math Operations/[-inf inf] to [-pi pi]  SystemSampleTime=-1
  yaw angle : Fcn  Expr=u(3)
  tag scope: ctrl1tau=global
  wires:
  [ctrl1Kd] -> Product2/1
  [ctrl1Ki] -> Product1/1
  [ctrl1Kp] -> Product/1
  Product1/1 -> Sum3/2
  Product/1 -> Sum3/1
  Product2/1 -> Sum1/2
  "[-inf inf] to [-pi pi]"/1 -> Mux/3
  Demux/3 -> "[-inf inf] to [-pi pi]"/1
  "[-inf inf] to [-pi pi]1"/1 -> Transposed rotation  matrix in yaw1/1
  yaw angle/1 -> "[-inf inf] to [-pi pi]1"/1  "psi"
  [ctrl1Reset] -> Integrator/2
  [nu] -> Product2/2
  Sum2/1 -> Demux/1
  Transposed rotation  matrix in yaw1/1 -> Product/2, Integrator/1
  Sum3/1 -> Sum1/1
  Integrator/1 -> Product1/2
  [eta] -> Sum2/2, yaw angle/1
  Sum1/1 -> [ctrl1tau]
  [setpoint] -> Sum2/1
  Demux/2 -> Mux/2
  Demux/1 -> Mux/1
  Mux/1 -> Transposed rotation  matrix in yaw1/2

== system NLPIDVersion2/Main Subsystems/Control/Nonlinear PID ==
  Auxilary functions g_q : Subsystem
  Auxiliary function g_s : Subsystem
  Control law : Subsystem
  R(psi) : Subsystem
  Update laws : Subsystem
  a_d : Subsystem
  e2 : Subsystem
  e_1 : Subsystem
  v_d : Subsystem
  zeta : Subsystem
  tag scope: q=global
  wires:
  Update laws/1(q) -> [q]
  Update laws/2(dot q) -> a_d/1(dot q)
  Update laws/3(dot s) -> a_d/2(dot s)

== system NLPIDVersion2/Main Subsystems/Control/PS3 u input control ==
  note: Manuel thruster control is intended for testing and flexing of thrusters and its signals
  note: Mapping PS3 signals to thruster settings:
      | - Y-position controls surge force of VSP
      | - X-positon controls sway force of VSP
      | - Left Analogstick controls port VSP
      | - Right Analogstick controls starboard VSP
      | - Postive values gives postive motions and vice versa
      | - R2 pressed gives postive yaw motion
      | - L2 pressed gives negative yaw motion
  Add : Sum  Inputs=|++
  Mux : Mux  Inputs=7
  PS3 u_{1..5} (5 alike) : Gain  ParameterDataType=fixdt(1, 16)  ParameterScaling=2^0  OutDataType=fixdt(1, 16)  OutScaling=2^0
  Subsystem : Subsystem
  tag scope: PS3tau=global, TCPS3=global
  wires:
  [PS3_AS_LX] -> PS3 u_2/1  "Left/Right position of Left Analogstick"
  [PS3_AS_LY] -> PS3 u_1/1  "Up/Down position of Left Analogstick"
  [PS3_AS_RY] -> PS3 u_3/1  "Up/Down position of Right Analogstick"
  [PS3_L2] -> Add/1  "L2 signal"
  [PS3_R2] -> Add/2  "R2 signal"
  [PS3_VSP_Speed] -> Mux/7  "VPS Speed"
  [PS3_BT_Power] -> Mux/6  "Bow Thruster Limit"
  Add/1 -> PS3 u_5/1  "Bow Thruster direction"
  Mux/1 -> Subsystem/1(u_act), [TCPS3]
  PS3 u_1/1 -> Mux/1  "u_1"
  PS3 u_2/1 -> Mux/2  "u_2"
  PS3 u_5/1 -> Mux/5  "u_5"
  PS3 u_4/1 -> Mux/4  "u_4"
  PS3 u_3/1 -> Mux/3  "u_3"
  Subsystem/1(tau) -> [PS3tau]
  [PS3_AS_RX] -> PS3 u_4/1  "Left/Right position of Right Analogstick"

== system NLPIDVersion2/Main Subsystems/Control/Thruster allocation ==
  Saturation : Saturate  UpperLimit=1.0  LowerLimit=-1.0
  VSP030 BT040 : Subsystem
  tau to f_act : Subsystem
  tag scope: TC=global, fact=global
  wires:
  [tau] -> tau to f_act/1(tau)
  tau to f_act/1(f_act) -> VSP030 BT040/1(f_act), [fact]
  VSP030 BT040/1(TC) -> Saturation/1
  Saturation/1 -> [TC]

== system NLPIDVersion2/Main Subsystems/Guidance/Line-Of-Sight Path-Following ==
  Heading : Subsystem
  Line-Of-Sight : Subsystem
  Path : Subsystem
  Speed assigment : Subsystem

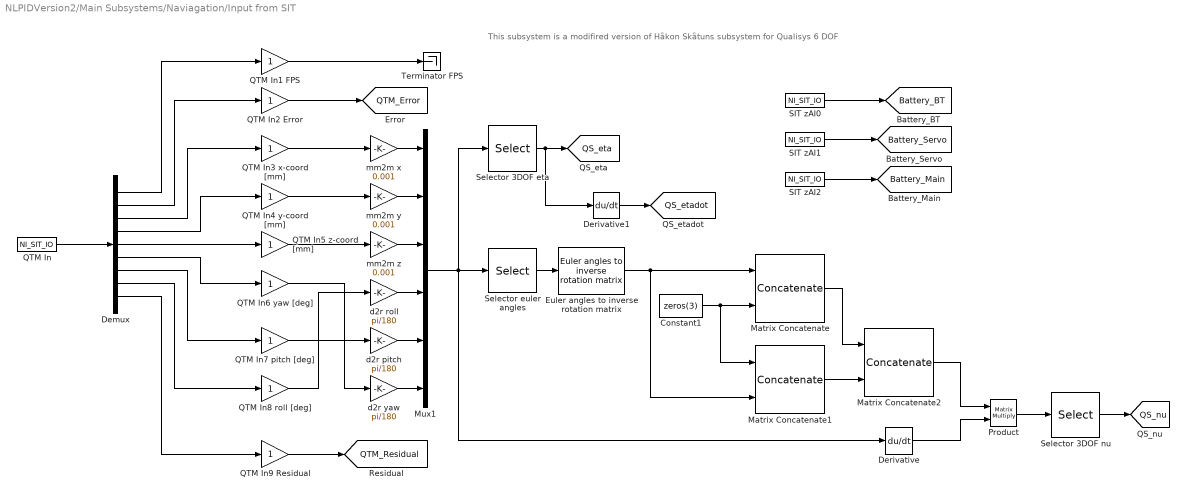
== system NLPIDVersion2/Main Subsystems/Naviagation/Input from SIT ==
  note: This subsystem is a modifired version of Håkon Skåtuns subsystem for Qualisys 6 DOF
  Constant1 : Constant  Value=zeros(3)
  Demux : Demux  Outputs=9
  Derivative : Derivative
  Derivative1 : Derivative
  Euler angles to inverse rotation matrix : marine_gnc/Models/ Kinematics/Euler angles to inverse rotation matrix  SystemSampleTime=-1
  Matrix Concatenate : Concatenate  Mode=Multidimensional array
  Matrix Concatenate1 : Concatenate  Mode=Multidimensional array
  Matrix Concatenate2 : Concatenate  Mode=Multidimensional array  ConcatenateDimension=2
  Mux1 : Mux  Inputs=6
  Product : Product  Multiplication=Matrix(*)  RndMeth=Zero
  QTM In : S-Function  Priority=1  FunctionName=NI_SIT_IO  Parameters=width dtype portnum stime stype btype  EnableBusSupport=off  mask(SIT Inport){portnum=1, width=9, stime=-1, dtype=auto, stype=auto, btype=1}
      mask prompts: portnum "Port number:"; width "Port dimensions (-1 for dynamically sized):"; stime "Sample time (-1 for inherited):"; dtype "Data type:"; stype "Signal type:"; btype "Block type:"
      mask help: Use this inport on any level of nested subsystems to allow the LabVIEW Simulation Interface Toolkit to map hardware to it.
      mask init:
      | NI_SIT_IO_init;
      settings: CopyFcn=NI_SIT_IO_callbacks(1);  DeleteFcn=NI_SIT_IO_callbacks(2);
      mask StyleString: edit,edit,edit,popup(auto|double|single|int8|uint8|int16|uint16|int32|uint32|boolean),popup(auto|real|complex),edit
      mask CallbackString: NI_SIT_IO_callbacks(3);|||NI_SIT_IO_callbacks(4);||
      mask TabNameString: Parameters,Parameters,Parameters,Parameters,Parameters,Parameters
      mask Display:
      | patch([-x x], [-y y], [.90980 .81960 .32156]);
      | plot([0 -x x 0], [rad -y y rad]);
      | fprintf('SIT%d', portnum);
  QTM In1 FPS : Gain  ParameterDataType=fixdt(1, 16)  ParameterScaling=2^0  OutDataType=fixdt(1, 16)  OutScaling=2^0
  QTM In2 Error : Gain  ParameterDataType=fixdt(1, 16)  ParameterScaling=2^0  OutDataType=fixdt(1, 16)  OutScaling=2^0
  QTM In3 x-coord [mm] : Gain  ParameterDataType=fixdt(1, 16)  ParameterScaling=2^0  OutDataType=fixdt(1, 16)  OutScaling=2^0
  QTM In4 y-coord [mm] : Gain  ParameterDataType=fixdt(1, 16)  ParameterScaling=2^0  OutDataType=fixdt(1, 16)  OutScaling=2^0
  QTM In5 z-coord [mm] : Gain  ParameterDataType=fixdt(1, 16)  ParameterScaling=2^0  OutDataType=fixdt(1, 16)  OutScaling=2^0
  QTM In6 yaw [deg] : Gain  ParameterDataType=fixdt(1, 16)  ParameterScaling=2^0  OutDataType=fixdt(1, 16)  OutScaling=2^0
  QTM In7 pitch [deg] : Gain  ParameterDataType=fixdt(1, 16)  ParameterScaling=2^0  OutDataType=fixdt(1, 16)  OutScaling=2^0
  QTM In8 roll [deg] : Gain  ParameterDataType=fixdt(1, 16)  ParameterScaling=2^0  OutDataType=fixdt(1, 16)  OutScaling=2^0
  QTM In9 Residual : Gain  ParameterDataType=fixdt(1, 16)  ParameterScaling=2^0  OutDataType=fixdt(1, 16)  OutScaling=2^0
  SIT zAI0 : S-Function  Priority=2  FunctionName=NI_SIT_IO  Parameters=width dtype portnum stime stype btype  EnableBusSupport=off  mask(SIT Inport){portnum=2, width=-1, stime=-1, dtype=auto, stype=auto, btype=1}
      mask prompts: portnum "Port number:"; width "Port dimensions (-1 for dynamically sized):"; stime "Sample time (-1 for inherited):"; dtype "Data type:"; stype "Signal type:"; btype "Block type:"
      mask help: Use this inport on any level of nested subsystems to allow the LabVIEW Simulation Interface Toolkit to map hardware to it.
      mask init:
      | NI_SIT_IO_init;
      settings: CopyFcn=NI_SIT_IO_callbacks(1);  DeleteFcn=NI_SIT_IO_callbacks(2);
      mask StyleString: edit,edit,edit,popup(auto|double|single|int8|uint8|int16|uint16|int32|uint32|boolean),popup(auto|real|complex),edit
      mask CallbackString: NI_SIT_IO_callbacks(3);|||NI_SIT_IO_callbacks(4);||
      mask TabNameString: Parameters,Parameters,Parameters,Parameters,Parameters,Parameters
      mask Display:
      | patch([-x x], [-y y], [.90980 .81960 .32156]);
      | plot([0 -x x 0], [rad -y y rad]);
      | fprintf('SIT%d', portnum);
  SIT zAI1 : S-Function  Priority=3  FunctionName=NI_SIT_IO  Parameters=width dtype portnum stime stype btype  EnableBusSupport=off  mask(SIT Inport){portnum=3, width=-1, stime=-1, dtype=auto, stype=auto, btype=1}
      mask prompts: portnum "Port number:"; width "Port dimensions (-1 for dynamically sized):"; stime "Sample time (-1 for inherited):"; dtype "Data type:"; stype "Signal type:"; btype "Block type:"
      mask help: Use this inport on any level of nested subsystems to allow the LabVIEW Simulation Interface Toolkit to map hardware to it.
      mask init:
      | NI_SIT_IO_init;
      settings: CopyFcn=NI_SIT_IO_callbacks(1);  DeleteFcn=NI_SIT_IO_callbacks(2);
      mask StyleString: edit,edit,edit,popup(auto|double|single|int8|uint8|int16|uint16|int32|uint32|boolean),popup(auto|real|complex),edit
      mask CallbackString: NI_SIT_IO_callbacks(3);|||NI_SIT_IO_callbacks(4);||
      mask TabNameString: Parameters,Parameters,Parameters,Parameters,Parameters,Parameters
      mask Display:
      | patch([-x x], [-y y], [.90980 .81960 .32156]);
      | plot([0 -x x 0], [rad -y y rad]);
      | fprintf('SIT%d', portnum);
  SIT zAI2 : S-Function  Priority=4  FunctionName=NI_SIT_IO  Parameters=width dtype portnum stime stype btype  EnableBusSupport=off  mask(SIT Inport){portnum=4, width=-1, stime=-1, dtype=auto, stype=auto, btype=1}
      mask prompts: portnum "Port number:"; width "Port dimensions (-1 for dynamically sized):"; stime "Sample time (-1 for inherited):"; dtype "Data type:"; stype "Signal type:"; btype "Block type:"
      mask help: Use this inport on any level of nested subsystems to allow the LabVIEW Simulation Interface Toolkit to map hardware to it.
      mask init:
      | NI_SIT_IO_init;
      settings: CopyFcn=NI_SIT_IO_callbacks(1);  DeleteFcn=NI_SIT_IO_callbacks(2);
      mask StyleString: edit,edit,edit,popup(auto|double|single|int8|uint8|int16|uint16|int32|uint32|boolean),popup(auto|real|complex),edit
      mask CallbackString: NI_SIT_IO_callbacks(3);|||NI_SIT_IO_callbacks(4);||
      mask TabNameString: Parameters,Parameters,Parameters,Parameters,Parameters,Parameters
      mask Display:
      | patch([-x x], [-y y], [.90980 .81960 .32156]);
      | plot([0 -x x 0], [rad -y y rad]);
      | fprintf('SIT%d', portnum);
  Selector 3DOF eta : Selector  InputPortWidth=6  IndexOptions=Index vector (dialog)  Indices=[1 2 6]  OutputSizes=1
  Selector 3DOF nu : Selector  InputPortWidth=6  IndexOptions=Index vector (dialog)  Indices=[1 2 6]  OutputSizes=1
  Selector euler angles : Selector  InputPortWidth=6  IndexOptions=Index vector (dialog)  Indices=[4 5 6]  OutputSizes=1
  Terminator FPS : Terminator
  d2r pitch : Gain  Gain=pi/180  ParameterDataType=fixdt(1, 16)  ParameterScaling=2^0  OutDataType=fixdt(1, 16)  OutScaling=2^0
  d2r roll : Gain  Gain=pi/180  ParameterDataType=fixdt(1, 16)  ParameterScaling=2^0  OutDataType=fixdt(1, 16)  OutScaling=2^0
  d2r yaw : Gain  Gain=pi/180  ParameterDataType=fixdt(1, 16)  ParameterScaling=2^0  OutDataType=fixdt(1, 16)  OutScaling=2^0
  mm2m x : Gain  Gain=0.001
  mm2m y : Gain  Gain=0.001
  mm2m z : Gain  Gain=0.001
  tag scope: Battery_BT=global, Battery_Main=global, Battery_Servo=global, QS_eta=global, QS_etadot=global, QS_nu=global, QTM_Error=global, QTM_Residual=global
  wires:
  SIT zAI2/1 -> [Battery_Main]
  SIT zAI1/1 -> [Battery_Servo]
  SIT zAI0/1 -> [Battery_BT]
  Derivative1/1 -> [QS_etadot]
  QTM In8 roll [deg]/1 -> d2r roll/1
  QTM In6 yaw [deg]/1 -> d2r yaw/1
  QTM In7 pitch [deg]/1 -> d2r pitch/1
  QTM In5 z-coord [mm]/1 -> mm2m z/1
  QTM In4 y-coord [mm]/1 -> mm2m y/1
  QTM In3 x-coord [mm]/1 -> mm2m x/1
  Demux/9 -> QTM In9 Residual/1
  Demux/8 -> QTM In8 roll [deg]/1
  Demux/7 -> QTM In7 pitch [deg]/1
  Demux/6 -> QTM In6 yaw [deg]/1
  Demux/5 -> QTM In5 z-coord [mm]/1
  Demux/4 -> QTM In4 y-coord [mm]/1
  Demux/3 -> QTM In3 x-coord [mm]/1
  Demux/2 -> QTM In2 Error/1
  Demux/1 -> QTM In1 FPS/1
  QTM In/1 -> Demux/1
  QTM In9 Residual/1 -> [QTM_Residual]
  QTM In2 Error/1 -> [QTM_Error]
  QTM In1 FPS/1 -> Terminator FPS/1
  Selector 3DOF nu/1 -> [QS_nu]
  Product/1 -> Selector 3DOF nu/1
  Selector euler angles/1 -> Euler angles to inverse rotation matrix/1
  d2r roll/1 -> Mux1/4
  d2r pitch/1 -> Mux1/5
  d2r yaw/1 -> Mux1/6
  mm2m x/1 -> Mux1/1
  mm2m y/1 -> Mux1/2
  mm2m z/1 -> Mux1/3
  Constant1/1 -> Matrix Concatenate1/1, Matrix Concatenate/2
  Derivative/1 -> Product/2
  Matrix Concatenate2/1 -> Product/1
  Matrix Concatenate1/1 -> Matrix Concatenate2/2
  Matrix Concatenate/1 -> Matrix Concatenate2/1
  Euler angles to inverse rotation matrix/1 -> Matrix Concatenate1/2, Matrix Concatenate/1
  Selector 3DOF eta/1 -> [QS_eta], Derivative1/1
  Mux1/1 -> Selector 3DOF eta/1, Derivative/1, Selector euler angles/1

== system NLPIDVersion2/Main Subsystems/Naviagation/Navigation Switch ==
  eta Switch : MultiPortSwitch  Inputs=2  zeroidx=on
  etadot Switch : MultiPortSwitch  Inputs=2  zeroidx=on
  nu Switch : MultiPortSwitch  Inputs=2  zeroidx=on
  tag scope: eta=global, etadot=global, nu=global
  wires:
  [controlInputSelector] -> eta Switch/1, nu Switch/1, etadot Switch/1
  [QS_eta] -> eta Switch/2
  [LS_eta] -> eta Switch/3
  [QS_nu] -> nu Switch/2
  [LS_nu] -> nu Switch/3
  [QS_etadot] -> etadot Switch/2
  [LS_etadot] -> etadot Switch/3
  eta Switch/1 -> [eta]
  nu Switch/1 -> [nu]
  etadot Switch/1 -> [etadot]

== system NLPIDVersion2/Main Subsystems/Plant/CSE1 actuator ==
  note: This subsystem is a modifired version of Håkon Skåtuns subsystem CSE1
  Thurster setting : Inport
  Enable : EnablePort  StatesWhenEnabling=reset
  Bow Thruster : Subsystem
  Demux : Demux  Outputs=7
  "Voith Schneider Propeller " : Subsystem
  wires:
  Thurster setting/1 -> Demux/1
  Demux/1 -> "Voith Schneider Propeller "/1(Port VSP y u_1)
  Demux/2 -> "Voith Schneider Propeller "/2(Port VSP x u_2)
  Demux/3 -> "Voith Schneider Propeller "/3(Starboard VSP y u_3)
  Demux/4 -> "Voith Schneider Propeller "/4(Starboard VSP x u_4)
  Demux/7 -> "Voith Schneider Propeller "/5(VSP Speed)
  Demux/5 -> Bow Thruster/1(Bow Thruster Direction u_5)
  Demux/6 -> Bow Thruster/2(Bow Thruster Power)

== system NLPIDVersion2/Main Subsystems/Plant/Linear Simulator ==
  tau : Inport
  M_inv : Inport  Port=2
  D_L : Inport  Port=3
  Reset : Inport  Port=4
  eta_0 : Inport  Port=5
  nu_0 : Inport  Port=6
  Enable : EnablePort  StatesWhenEnabling=reset
  Linear Vessel Dynamics : Subsystem
  eta_hil : Outport
  nu_hil : Outport  Port=2
  etadot_hil : Outport  Port=3
  wires:
  tau/1 -> Linear Vessel Dynamics/1(tau)
  Linear Vessel Dynamics/1(eta) -> eta_hil/1
  Linear Vessel Dynamics/2(nu) -> nu_hil/1
  Linear Vessel Dynamics/3(etadot) -> etadot_hil/1
  M_inv/1 -> Linear Vessel Dynamics/2(M_inv)
  D_L/1 -> Linear Vessel Dynamics/3(D_L)
  Reset/1 -> Linear Vessel Dynamics/4(Reset)
  eta_0/1 -> Linear Vessel Dynamics/5(eta_0)
  nu_0/1 -> Linear Vessel Dynamics/6(nu_0)

== system NLPIDVersion2/Main Subsystems/Plant/Thruster setting workaround ==
  note: 0 - Direct PS3
      | else TC from Control subsystem
  TC : Inport  OutDataType=fixdt(1, 16)  OutScaling=2^0
  Saturation : Saturate  UpperLimit=1  LowerLimit=0  OutDataType=fixdt(1, 16)  OutScaling=2^0
  tau Switch : MultiPortSwitch  Inputs=2  zeroidx=on
  tag scope: ThrusterSetting=global
  wires:
  tau Switch/1 -> [ThrusterSetting]
  TC/1 -> tau Switch/3
  [TCPS3] -> tau Switch/2
  [controlModeSelector] -> Saturation/1
  Saturation/1 -> tau Switch/1

== system NLPIDVersion2/Main Subsystems/Plant/saturation ==
  tau : Inport  OutDataType=sfix(16)  OutScaling=2^0
  Demux : Demux  Outputs=3
  Mux1 : Mux  Inputs=3
  Saturation : Saturate  UpperLimit=3  LowerLimit=-2.6  OutDataType=fixdt(1, 16)  OutScaling=2^0
  Saturation1 : Saturate  UpperLimit=3  LowerLimit=-3.5  OutDataType=fixdt(1, 16)  OutScaling=2^0
  Saturation2 : Saturate  UpperLimit=1.6  LowerLimit=-1.5  OutDataType=fixdt(1, 16)  OutScaling=2^0
  plant tau_surge : Gain  ParameterDataType=fixdt(1, 16)  ParameterScaling=2^0  OutDataType=fixdt(1, 16)  OutScaling=2^0
  plant tau_sway : Gain  ParameterDataType=fixdt(1, 16)  ParameterScaling=2^0  OutDataType=fixdt(1, 16)  OutScaling=2^0
  plant tau_yaw : Gain  ParameterDataType=fixdt(1, 16)  ParameterScaling=2^0  OutDataType=fixdt(1, 16)  OutScaling=2^0
  sat_tau : Outport  OutDataType=sfix(16)  OutScaling=2^0
  wires:
  Mux1/1 -> sat_tau/1
  tau/1 -> Demux/1
  Saturation/1 -> plant tau_surge/1
  Demux/1 -> Saturation/1
  Demux/2 -> Saturation1/1
  Saturation1/1 -> plant tau_sway/1
  plant tau_surge/1 -> Mux1/1
  plant tau_sway/1 -> Mux1/2
  Demux/3 -> Saturation2/1
  Saturation2/1 -> plant tau_yaw/1
  plant tau_yaw/1 -> Mux1/3

== system NLPIDVersion2/Main Subsystems/Control/Nonlinear PID/Auxilary functions g_q ==
  g_q eq : Subsystem
  g_q^q eq : Subsystem
  g_q^s eq : Subsystem
  g_q^t eq : Subsystem
  tag scope: gq=global, gq_q=global, gq_s=global, gq_t=global
  wires:
  [fq_t] -> g_q^t eq/2(f_q^t)
  g_q^t eq/1(g_q^t) -> [gq_t]
  [psiLOS_qs] -> g_q^s eq/4(psi_los^qs)
  [fq_s] -> g_q^s eq/3(f_q^s)
  g_q^s eq/1(g_q^s) -> [gq_s]
  g_q^q eq/1(g_q^q) -> [gq_q]
  [psiLOS_q_2] -> g_q^q eq/4(psi_los^q^2)
  [fq_q] -> g_q^q eq/3(f_q^q)
  [fq] -> g_q^s eq/1(f_q), g_q^q eq/1(f_q), g_q eq/1(f_q)
  [psiLOS_q] -> g_q^t eq/1(psi_los^q), g_q^s eq/2(psi_los^q), g_q^q eq/2(psi_los^q), g_q eq/2(psi_los^q)
  g_q eq/1(g_q) -> [gq]
